simulink model "full_maneuver_platoon"  (R2022a)
settings: Solver=ode23t  StartTime=0.0  StopTime=300  FixedStep=0.1  MaxStep=0.01  RelTol=1e-3
InitFcn:
  | totalVehicles = 7;
  | if exist('vehStatesBus', 'var')==0
  | load vehBuses
  | end
  | if exist('vehErrorsBus', 'var')==0
  | load vehBuses
  | end
libraries: simulink x80, powerlib_meascontrol x16, autolibshared x7, dspsigops x4
(part 3 of 9)

== system full_maneuver_platoon/p1/CACC origin lane ==
  ego : Inport
  leader : Inport  Port=2
  referenceSpeed : Inport  Port=3
  leaderChange : Inport  Port=4
  extraSpaceFlag : Inport  Port=5
  Bus Selector : BusSelector  OutputSignals=u
  Compute Errors : Subsystem
  Constant : Constant  Value=0
  Constant1 : Constant  Value=1.2*freeFlowVel
  Define Desired Distance : Subsystem
  Demux : Demux  Outputs=2
  NOT : Logic  Operator=NOT  IconShape=distinctive  AllPortsSameDT=off  OutDataTypeStr=boolean
  NOT1 : Logic  Operator=NOT  IconShape=distinctive  AllPortsSameDT=off  OutDataTypeStr=boolean
  Rate Limiter : RateLimiter  RisingSlewLimit=maxJerk  FallingSlewLimit=minJerk  SampleTimeMode=inherited
  Rate Limiter1 : RateLimiter  RisingSlewLimit=maxComfJerk  FallingSlewLimit=minComfJerk  SampleTimeMode=inherited
  Switch : Switch  Criteria=u2 > Threshold  SaturateOnIntegerOverflow=off  InputSameDT=off
  Switch1 : Switch  Criteria=u2 > Threshold  SaturateOnIntegerOverflow=off  InputSameDT=off
  Veh Following : Subsystem  TreatAsAtomicUnit=on
  Velocity Control : Subsystem  TreatAsAtomicUnit=on
  Velocity Error : Subsystem
  comf saturation : Saturate  UpperLimit=maxComfAccel  LowerLimit=minComfAccel
  errorScope : Scope  NumInputPorts=2
  safe saturation : Saturate  UpperLimit=maxAcceleration  LowerLimit=minAcceleration
  switch free flow : Subsystem
  veh foll state : Scope  NumInputPorts=2
  errors : Outport
  gap : Outport  Port=2
  u : Outport  Port=3
  real veh foll state : Outport  Port=4
  wires:
  Compute Errors/3("gap ") -> gap/1, switch free flow/3(gap)
  Compute Errors/1(errors) -> Veh Following/1(errors), Demux/1, errors/1, switch free flow/1(errors)
  Switch1/1 -> u/1
  Demux/1 -> errorScope/1
  Demux/2 -> errorScope/2
  NOT1/1 -> Velocity Control/3(integralReset)
  NOT/1 -> Velocity Error/3(filterReset)
  Constant1/1 -> switch free flow/6(vRef)
  extraSpaceFlag/1 -> Define Desired Distance/1(extraSpaceFlag)
  switch free flow/1(inRange) -> NOT/1, NOT1/1, real veh foll state/1, veh foll state/1, Switch/2, Veh Following/5(inRange)
  Velocity Error/1(ev) -> Velocity Control/1(ev)
  Velocity Error/2(ea) -> Velocity Control/2(ea)
  leaderChange/1 -> Veh Following/4(leaderChange)
  Veh Following/1(u) -> Switch/1
  Constant/1 -> Compute Errors/5(velFilterReset)
  leader/1 -> Compute Errors/2(leader)
  comf saturation/1 -> Rate Limiter1/1
  safe saturation/1 -> Rate Limiter/1
  Rate Limiter/1 -> Switch1/1  "sat(u)"
  Switch/1 -> comf saturation/1, safe saturation/1, veh foll state/2
  Rate Limiter1/1 -> Switch1/3  "sat(u)"
  ego/1 -> Velocity Error/1(ego), Bus Selector/1, Compute Errors/1(ego)
  Velocity Control/1(u) -> Switch/3
  referenceSpeed/1 -> Velocity Error/2(velRef)
  Compute Errors/4(unsafeFlag) -> Switch1/2
  Bus Selector/1 -> Veh Following/3(realInput)  "<u>"
  Compute Errors/2(errorsDot) -> switch free flow/2(errorsDot), Veh Following/2(errorsDot)
  Define Desired Distance/1(h) -> switch free flow/4(h), Compute Errors/3(h)
  Define Desired Distance/2(d0) -> switch free flow/5(d0), Compute Errors/4(d0)

== system full_maneuver_platoon/p1/Check if Gap is Closed ==
  In1 : Inport
  AND : Logic  Inputs=1  IconShape=distinctive  AllPortsSameDT=off  OutDataTypeStr=boolean
  Abs2 : Abs  SaturateOnIntegerOverflow=off
  Compare To Constant2 : simulink/Logic and Bit Operations/Compare To Constant  relop=<=  const=1  OutDataTypeStr=boolean
  Mux : Mux  Inputs=2
  Transport Delay2 : TransportDelay
  Out1 : Outport
  wires:
  Transport Delay2/1 -> Mux/1
  Abs2/1 -> Compare To Constant2/1
  Compare To Constant2/1 -> AND/1
  Mux/1 -> Abs2/1
  In1/1 -> Transport Delay2/1, Mux/2
  AND/1 -> Out1/1

== system full_maneuver_platoon/p1/Find Leader ==
  ego : Inport
  all : Inport  Port=2
  canStartLaneChange : Inport  Port=3
  laneChangeDone : Inport  Port=4
  Detect Change : simulink/Logic and Bit Operations/Detect Change  vinit=0  OutDataTypeStr=boolean
  NOT : Logic  Operator=NOT  IconShape=distinctive  AllPortsSameDT=off  OutDataTypeStr=boolean
  OR : Logic  Operator=OR  IconShape=distinctive  AllPortsSameDT=off  OutDataTypeStr=boolean
  Selector : Selector  InputPortWidth=totalVehicles+1  IndexOptions=Index vector (port)  Indices=[1]  OutputSizes=1
  Subsystem : Subsystem
  Vector Concatenate : Concatenate
  farAwayVeh : Subsystem
  realLeaderIdx : Scope
  leader : Outport  VectorParamsAs1DForOutWhenUnconnected=off
  leaderChange : Outport  Port=2  VectorParamsAs1DForOutWhenUnconnected=off
  wires:
  Vector Concatenate/1 -> Selector/1
  farAwayVeh/1(Out1) -> Vector Concatenate/2
  Subsystem/1(idx) -> Detect Change/1, Selector/2, realLeaderIdx/1
  NOT/1 -> OR/1
  canStartLaneChange/1 -> NOT/1
  OR/1 -> Subsystem/Enable  "isLaneChanging"
  all/1 -> Subsystem/2(all), Vector Concatenate/1
  ego/1 -> farAwayVeh/1(ego), Subsystem/1(ego)
  laneChangeDone/1 -> OR/2
  Selector/1 -> leader/1
  Detect Change/1 -> leaderChange/1

== system full_maneuver_platoon/p1/Lane Change Strategy ==
  note: 1) Add Subsystem or Model blocks as valid variant choices.
      | 2) You cannot connect blocks at this level. At simulation, connectivity is automatically
      | determined, based on the active variant and port name matching.
  gapRequest : Inport
  lcFlag : Inport  Port=2
  positionInPlatoon : Inport  Port=3
  platoonStates : Inport  Port=4
  isLaneChangeSafe : Inport  Port=5
  isLaneChangeDone : Inport  Port=6
  isGapClosed : Inport  Port=7
  realCACCstate : Inport  Port=8
  Strategy 1: synchronous : Subsystem  VariantControl=synchronous
  Strategy 2: leader first : Subsystem  VariantControl=leaderFirst
  Strategy 3: last first : Subsystem  VariantControl=lastFirst
  Strategy 4: leader first invert : Subsystem  VariantControl=leaderFirstInvert
  maneuverState : Outport
  mustIncreaseGap : Outport  Port=2
  canStartLaneChange : Outport  Port=3
  hasVirtualLeader : Outport  Port=4
  virtualLeaderIdx : Outport  Port=5
  virtualFollowerIdx : Outport  Port=6

== system full_maneuver_platoon/p1/Lateral Control ==
  measuredStates : Inport
  yRef : Inport  Port=2
  Demux2 : Demux
  Full State Observer : Subsystem  Commented=on
  Gain : Gain  Gain=5
  Gain1 : Gain  Gain=Klat  Multiplication=Matrix(K*u)
  Integrator : Integrator  InitialCondition=y0
  Pad : dspsigops/Pad  padAlong=Columns  dimsToPad=1  valSrc=Specify via dialog  padVal=0  spec=Output size  padNumOutRowsSpecMethod=User-specified  numOutRows=4  padNumOutColsSpecMethod=User-specified  numOutCols=1  isVarDimsMode=off  padBeginning=0  padEnd=0  outSizeMode=User-specified  outSize=1  padSigAt=End  trunc_flag=None  roundingMode=Floor  overflowMode=off  truncOrWrapMode=Truncate  wrap_flag=None
      settings: SourceProductBaseCode=DS
  Rate Limiter : RateLimiter  RisingSlewLimit=maxDeltaDot  FallingSlewLimit=-maxDeltaDot  SampleTimeMode=inherited
  Saturation : Saturate  UpperLimit=maxDelta  LowerLimit=-maxDelta
  Saturation1 : Saturate  UpperLimit=2  LowerLimit=-2
  Scope : Scope  NumInputPorts=4
  Scope1 : Scope  NumInputPorts=2
  Selector : Selector  InputPortWidth=4  IndexOptions=Index vector (dialog)  Indices=[1]  OutputSizes=1
  Sum : Sum  Inputs=|+-
  Sum2 : Sum  Inputs=|+-
  delta : Outport  VectorParamsAs1DForOutWhenUnconnected=off
  ey : Outport  Port=2  VectorParamsAs1DForOutWhenUnconnected=off
  wires:
  Selector/1 -> ey/1
  Saturation1/1 -> Integrator/1
  Gain/1 -> Saturation1/1
  measuredStates/1 -> Sum/2, Demux2/1, Full State Observer/1(measuredOutputs)  "estStates"
  yRef/1 -> Sum2/1
  Demux2/3 -> Scope/3
  Saturation/1 -> Rate Limiter/1
  Sum2/1 -> Gain/1
  Demux2/2 -> Scope/2
  Demux2/4 -> Scope/4
  Pad/1 -> Sum/1
  Sum/1 -> Gain1/1, Selector/1
  Gain1/1 -> Saturation/1, Scope1/2
  Integrator/1 -> Pad/1, Sum2/2
  Demux2/1 -> Scope/1
  Rate Limiter/1 -> delta/1, Scope1/1, Full State Observer/2(delta)  "delta"

== system full_maneuver_platoon/p1/Subsystem ==
  real u : Inport
  real CACC state : Inport  Port=2
  virtual u : Inport  Port=3
  virtual CACC active : Inport  Port=4
  AND : Logic  IconShape=distinctive  AllPortsSameDT=off  OutDataTypeStr=boolean
  Min : MinMax  Inputs=2
  NOT : Logic  Operator=NOT  IconShape=distinctive  AllPortsSameDT=off  OutDataTypeStr=boolean
  Switch : Switch  Criteria=u2 ~= 0  SaturateOnIntegerOverflow=off  InputSameDT=off
  possible inputs : Scope  NumInputPorts=2
  u : Outport
  wires:
  real u/1 -> Min/1, possible inputs/1
  virtual u/1 -> Switch/1, Min/2, possible inputs/2
  Min/1 -> Switch/3
  real CACC state/1 -> NOT/1
  NOT/1 -> AND/1
  virtual CACC active/1 -> AND/2
  AND/1 -> Switch/2
  Switch/1 -> u/1

== system full_maneuver_platoon/p1/Virtual Follower Error ==
  all : Inport
  virtualFollowerIdx : Inport  Port=2
  Enable : EnablePort
  Bus Selector : BusSelector  OutputSignals=egVirtual,evVirtual
  Mux : Mux  Inputs=2
  Scope : Scope
  Selector1 : Selector  InputPortWidth=totalVehicles  IndexOptions=Index vector (port)  Indices=[1]  OutputSizes=1
  virtual follower scope : Scope  NumInputPorts=2
  virtualError : Outport  InitialOutput=[0; 0]
  wires:
  all/1 -> Selector1/1
  virtualFollowerIdx/1 -> Scope/1, Selector1/2
  Mux/1 -> virtualError/1
  Selector1/1 -> Bus Selector/1
  Bus Selector/1 -> Mux/1, virtual follower scope/1  "<egVirtual>"
  Bus Selector/2 -> Mux/2, virtual follower scope/2  "<evVirtual>"

== system full_maneuver_platoon/p1/lateral steady state ==
  e : Inport
  AND : Logic  IconShape=distinctive  AllPortsSameDT=off  OutDataTypeStr=boolean
  Abs2 : Abs  SaturateOnIntegerOverflow=off
  Compare To Constant2 : simulink/Logic and Bit Operations/Compare To Constant  relop=<=  const=0.1  OutDataTypeStr=boolean
  Demux : Demux  Outputs=2
  Mux : Mux  Inputs=2
  Transport Delay2 : TransportDelay
  ssFlag : Outport  VectorParamsAs1DForOutWhenUnconnected=off
  wires:
  Demux/2 -> AND/2
  Mux/1 -> Abs2/1
  Compare To Constant2/1 -> Demux/1
  AND/1 -> ssFlag/1
  Transport Delay2/1 -> Mux/1
  Demux/1 -> AND/1
  Abs2/1 -> Compare To Constant2/1
  e/1 -> Mux/2, Transport Delay2/1

== system full_maneuver_platoon/p1/safeErrors ==
  errors : Inport
  AND : Logic  Inputs=1  IconShape=distinctive  AllPortsSameDT=off  OutDataTypeStr=boolean
  Compare To Constant4 : simulink/Logic and Bit Operations/Compare To Constant  relop=>=  const=-0.1  OutDataTypeStr=boolean
  safetyFlag : Outport  VectorParamsAs1DForOutWhenUnconnected=off
  wires:
  Compare To Constant4/1 -> AND/1
  errors/1 -> Compare To Constant4/1
  AND/1 -> safetyFlag/1

== system full_maneuver_platoon/p1/safeErrors1 ==
  errors : Inport
  AND : Logic  Inputs=1  IconShape=distinctive  AllPortsSameDT=off  OutDataTypeStr=boolean
  Compare To Constant4 : simulink/Logic and Bit Operations/Compare To Constant  relop=>=  const=-0.3  OutDataTypeStr=boolean
  safetyFlag : Outport  VectorParamsAs1DForOutWhenUnconnected=off
  wires:
  Compare To Constant4/1 -> AND/1
  errors/1 -> Compare To Constant4/1
  AND/1 -> safetyFlag/1

== system full_maneuver_platoon/p1/safeErrors2 ==
  errors : Inport
  AND : Logic  Inputs=1  IconShape=distinctive  AllPortsSameDT=off  OutDataTypeStr=boolean
  Compare To Constant4 : simulink/Logic and Bit Operations/Compare To Constant  relop=>=  const=-0.3  OutDataTypeStr=boolean
  safetyFlag : Outport  VectorParamsAs1DForOutWhenUnconnected=off
  wires:
  Compare To Constant4/1 -> AND/1
  AND/1 -> safetyFlag/1
  errors/1 -> Compare To Constant4/1

== system full_maneuver_platoon/p1/states routing ==
  delta : Inport
  Info : Inport  Port=2
  u : Inport  Port=3
  realError : Inport  Port=4
  virtualError : Inport  Port=5
  IatError : Inport  Port=6
  Bus Creator : BusCreator  Inputs=12  OutDataTypeStr=Bus: vehStatesBus  NonVirtualBus=on
      settings: InheritFromInputs=off
  Bus Selector : BusSelector  OutputSignals=BdyFrm.Cg.Vel.ydot,BdyFrm.Cg.AngVel.r,InertFrm.RearAxl.Disp.X,InertFrm.Cg.Disp.Y,InertFrm.RearAxl.Vel.Xdot,BdyFrm.Cg.Acc.xddot,InertFrm.Cg.Ang.psi
  Demux : Demux  Outputs=2
  Demux1 : Demux  Outputs=2
  Mux : Mux
  latStates : Outport
  observedStates : Outport  Port=2
  wires:
  Info/1 -> Bus Selector/1
  Bus Selector/3 -> Bus Creator/1  "<X>"
  Bus Selector/4 -> Bus Creator/2, Mux/1  "<Y>"
  Bus Selector/5 -> Bus Creator/3  "<Xdot>"
  Bus Selector/6 -> Bus Creator/4  "<xddot>"
  Bus Selector/7 -> Mux/3, Bus Creator/5  "<psi>"
  u/1 -> Bus Creator/6
  delta/1 -> Bus Creator/7
  Mux/1 -> latStates/1
  Bus Selector/1 -> Mux/2  "<ydot>"
  Bus Selector/2 -> Mux/4  "<r>"
  Bus Creator/1 -> observedStates/1
  realError/1 -> Demux/1
  virtualError/1 -> Demux1/1
  Demux/1 -> Bus Creator/8
  Demux/2 -> Bus Creator/9
  Demux1/1 -> Bus Creator/10
  Demux1/2 -> Bus Creator/11
  IatError/1 -> Bus Creator/12

== system full_maneuver_platoon/p1/steadyState ==
  u : Inport
  AND : Logic  Inputs=1  IconShape=distinctive  AllPortsSameDT=off  OutDataTypeStr=boolean
  Abs2 : Abs  SaturateOnIntegerOverflow=off
  Compare To Constant2 : simulink/Logic and Bit Operations/Compare To Constant  relop=<=  const=0.2  OutDataTypeStr=boolean
  Mux : Mux  Inputs=2
  Transport Delay2 : TransportDelay
  ssFlag : Outport  VectorParamsAs1DForOutWhenUnconnected=off
  wires:
  Compare To Constant2/1 -> AND/1
  u/1 -> Transport Delay2/1, Mux/2
  Abs2/1 -> Compare To Constant2/1
  Transport Delay2/1 -> Mux/1
  AND/1 -> ssFlag/1
  Mux/1 -> Abs2/1

== system full_maneuver_platoon/p2/CACC destination lane ==
  ego : Inport
  all : Inport  Port=2
  virtualLeaderIdx : Inport  Port=3
  extraSpace : Inport  Port=4
  Enable : EnablePort
  Demux : Demux  Outputs=2
  Detect Change : simulink/Logic and Bit Operations/Detect Change  vinit=0  OutDataTypeStr=boolean
  Scope virtualLeaderIdx : Scope
  Selector : Selector  InputPortWidth=totalVehicles  IndexOptions=Index vector (port)  Indices=[1]  OutputSizes=1
  Subsystem : Subsystem  Commented=through
  Virtual Vehicle Following : Subsystem  TreatAsAtomicUnit=on
  virtual error scope : Scope  NumInputPorts=2
  u : Outport  OutputWhenDisabled=reset  InitialOutput=maxAcceleration+1
  virtualErrors : Outport  Port=2  InitialOutput=[0; 0]
  virtualGap : Outport  Port=3  InitialOutput=[0]
  wires:
  Subsystem/1(u smooth) -> u/1
  virtualLeaderIdx/1 -> Detect Change/1, Selector/2, Scope virtualLeaderIdx/1
  all/1 -> Selector/1
  Demux/2 -> virtual error scope/2
  Demux/1 -> virtual error scope/1
  ego/1 -> Virtual Vehicle Following/1(ego)
  Virtual Vehicle Following/1(u) -> Subsystem/1(u)
  Virtual Vehicle Following/3(virtualGap) -> virtualGap/1
  Virtual Vehicle Following/2(virtualErrors) -> virtualErrors/1, Demux/1
  Detect Change/1 -> Virtual Vehicle Following/3(leaderChange)
  Selector/1 -> Virtual Vehicle Following/2(virtualLeader)
  extraSpace/1 -> Virtual Vehicle Following/4(extraSpaceFlag)

== system full_maneuver_platoon/p2/CACC origin lane ==
  ego : Inport
  leader : Inport  Port=2
  referenceSpeed : Inport  Port=3
  leaderChange : Inport  Port=4
  extraSpaceFlag : Inport  Port=5
  Bus Selector : BusSelector  OutputSignals=u
  Compute Errors : Subsystem
  Constant : Constant  Value=0
  Constant1 : Constant  Value=1.2*freeFlowVel
  Define Desired Distance : Subsystem
  Demux : Demux  Outputs=2
  NOT : Logic  Operator=NOT  IconShape=distinctive  AllPortsSameDT=off  OutDataTypeStr=boolean
  NOT1 : Logic  Operator=NOT  IconShape=distinctive  AllPortsSameDT=off  OutDataTypeStr=boolean
  Rate Limiter : RateLimiter  RisingSlewLimit=maxJerk  FallingSlewLimit=minJerk  SampleTimeMode=inherited
  Rate Limiter1 : RateLimiter  RisingSlewLimit=maxComfJerk  FallingSlewLimit=minComfJerk  SampleTimeMode=inherited
  Switch : Switch  Criteria=u2 > Threshold  SaturateOnIntegerOverflow=off  InputSameDT=off
  Switch1 : Switch  Criteria=u2 > Threshold  SaturateOnIntegerOverflow=off  InputSameDT=off
  Veh Following : Subsystem  TreatAsAtomicUnit=on
  Velocity Control : Subsystem  TreatAsAtomicUnit=on
  Velocity Error : Subsystem
  comf saturation : Saturate  UpperLimit=maxComfAccel  LowerLimit=minComfAccel
  errorScope : Scope  NumInputPorts=2
  safe saturation : Saturate  UpperLimit=maxAcceleration  LowerLimit=minAcceleration
  switch free flow : Subsystem
  veh foll state : Scope  NumInputPorts=2
  errors : Outport
  gap : Outport  Port=2
  u : Outport  Port=3
  real veh foll state : Outport  Port=4
  wires:
  Define Desired Distance/2(d0) -> Compute Errors/4(d0), switch free flow/5(d0)
  Define Desired Distance/1(h) -> Compute Errors/3(h), switch free flow/4(h)
  Compute Errors/2(errorsDot) -> Veh Following/2(errorsDot), switch free flow/2(errorsDot)
  Bus Selector/1 -> Veh Following/3(realInput)  "<u>"
  Compute Errors/4(unsafeFlag) -> Switch1/2
  referenceSpeed/1 -> Velocity Error/2(velRef)
  Velocity Control/1(u) -> Switch/3
  ego/1 -> Compute Errors/1(ego), Bus Selector/1, Velocity Error/1(ego)
  Rate Limiter1/1 -> Switch1/3  "sat(u)"
  Switch/1 -> veh foll state/2, safe saturation/1, comf saturation/1
  Rate Limiter/1 -> Switch1/1  "sat(u)"
  safe saturation/1 -> Rate Limiter/1
  comf saturation/1 -> Rate Limiter1/1
  leader/1 -> Compute Errors/2(leader)
  Constant/1 -> Compute Errors/5(velFilterReset)
  Veh Following/1(u) -> Switch/1
  leaderChange/1 -> Veh Following/4(leaderChange)
  Velocity Error/2(ea) -> Velocity Control/2(ea)
  Velocity Error/1(ev) -> Velocity Control/1(ev)
  switch free flow/1(inRange) -> Veh Following/5(inRange), Switch/2, veh foll state/1, real veh foll state/1, NOT1/1, NOT/1
  extraSpaceFlag/1 -> Define Desired Distance/1(extraSpaceFlag)
  Constant1/1 -> switch free flow/6(vRef)
  NOT/1 -> Velocity Error/3(filterReset)
  NOT1/1 -> Velocity Control/3(integralReset)
  Demux/2 -> errorScope/2
  Demux/1 -> errorScope/1
  Switch1/1 -> u/1
  Compute Errors/1(errors) -> switch free flow/1(errors), errors/1, Demux/1, Veh Following/1(errors)
  Compute Errors/3("gap ") -> switch free flow/3(gap), gap/1

== system full_maneuver_platoon/p2/Check if Gap is Closed ==
  In1 : Inport
  AND : Logic  Inputs=1  IconShape=distinctive  AllPortsSameDT=off  OutDataTypeStr=boolean
  Abs2 : Abs  SaturateOnIntegerOverflow=off
  Compare To Constant2 : simulink/Logic and Bit Operations/Compare To Constant  relop=<=  const=1  OutDataTypeStr=boolean
  Mux : Mux  Inputs=2
  Transport Delay2 : TransportDelay
  Out1 : Outport
  wires:
  AND/1 -> Out1/1
  In1/1 -> Mux/2, Transport Delay2/1
  Mux/1 -> Abs2/1
  Compare To Constant2/1 -> AND/1
  Abs2/1 -> Compare To Constant2/1
  Transport Delay2/1 -> Mux/1

== system full_maneuver_platoon/p2/Find Leader ==
  ego : Inport
  all : Inport  Port=2
  canStartLaneChange : Inport  Port=3
  laneChangeDone : Inport  Port=4
  Detect Change : simulink/Logic and Bit Operations/Detect Change  vinit=0  OutDataTypeStr=boolean
  NOT : Logic  Operator=NOT  IconShape=distinctive  AllPortsSameDT=off  OutDataTypeStr=boolean
  OR : Logic  Operator=OR  IconShape=distinctive  AllPortsSameDT=off  OutDataTypeStr=boolean
  Selector : Selector  InputPortWidth=totalVehicles+1  IndexOptions=Index vector (port)  Indices=[1]  OutputSizes=1
  Subsystem : Subsystem
  Vector Concatenate : Concatenate
  farAwayVeh : Subsystem
  realLeaderIdx : Scope
  leader : Outport  VectorParamsAs1DForOutWhenUnconnected=off
  leaderChange : Outport  Port=2  VectorParamsAs1DForOutWhenUnconnected=off
  wires:
  Detect Change/1 -> leaderChange/1
  Selector/1 -> leader/1
  laneChangeDone/1 -> OR/2
  ego/1 -> Subsystem/1(ego), farAwayVeh/1(ego)
  all/1 -> Vector Concatenate/1, Subsystem/2(all)
  OR/1 -> Subsystem/Enable  "isLaneChanging"
  canStartLaneChange/1 -> NOT/1
  NOT/1 -> OR/1
  Subsystem/1(idx) -> realLeaderIdx/1, Selector/2, Detect Change/1
  farAwayVeh/1(Out1) -> Vector Concatenate/2
  Vector Concatenate/1 -> Selector/1

== system full_maneuver_platoon/p2/Lane Change Strategy ==
  note: 1) Add Subsystem or Model blocks as valid variant choices.
      | 2) You cannot connect blocks at this level. At simulation, connectivity is automatically
      | determined, based on the active variant and port name matching.
  gapRequest : Inport
  lcFlag : Inport  Port=2
  positionInPlatoon : Inport  Port=3
  platoonStates : Inport  Port=4
  isLaneChangeSafe : Inport  Port=5
  isLaneChangeDone : Inport  Port=6
  isGapClosed : Inport  Port=7
  realCACCstate : Inport  Port=8
  Strategy 1: synchronous : Subsystem  VariantControl=synchronous
  Strategy 2: leader first : Subsystem  VariantControl=leaderFirst
  Strategy 3: last first : Subsystem  VariantControl=lastFirst
  Strategy 4: leader first invert : Subsystem  VariantControl=leaderFirstInvert
  maneuverState : Outport
  mustIncreaseGap : Outport  Port=2
  canStartLaneChange : Outport  Port=3
  hasVirtualLeader : Outport  Port=4
  virtualLeaderIdx : Outport  Port=5
  virtualFollowerIdx : Outport  Port=6

== system full_maneuver_platoon/p2/Lateral Control ==
  measuredStates : Inport
  yRef : Inport  Port=2
  Demux2 : Demux
  Full State Observer : Subsystem  Commented=on
  Gain : Gain  Gain=5
  Gain1 : Gain  Gain=Klat  Multiplication=Matrix(K*u)
  Integrator : Integrator  InitialCondition=y0
  Pad : dspsigops/Pad  padAlong=Columns  dimsToPad=1  valSrc=Specify via dialog  padVal=0  spec=Output size  padNumOutRowsSpecMethod=User-specified  numOutRows=4  padNumOutColsSpecMethod=User-specified  numOutCols=1  isVarDimsMode=off  padBeginning=0  padEnd=0  outSizeMode=User-specified  outSize=1  padSigAt=End  trunc_flag=None  roundingMode=Floor  overflowMode=off  truncOrWrapMode=Truncate  wrap_flag=None
      settings: SourceProductBaseCode=DS
  Rate Limiter : RateLimiter  RisingSlewLimit=maxDeltaDot  FallingSlewLimit=-maxDeltaDot  SampleTimeMode=inherited
  Saturation : Saturate  UpperLimit=maxDelta  LowerLimit=-maxDelta
  Saturation1 : Saturate  UpperLimit=2  LowerLimit=-2
  Scope : Scope  NumInputPorts=4
  Scope1 : Scope  NumInputPorts=2
  Selector : Selector  InputPortWidth=4  IndexOptions=Index vector (dialog)  Indices=[1]  OutputSizes=1
  Sum : Sum  Inputs=|+-
  Sum2 : Sum  Inputs=|+-
  delta : Outport  VectorParamsAs1DForOutWhenUnconnected=off
  ey : Outport  Port=2  VectorParamsAs1DForOutWhenUnconnected=off
  wires:
  Rate Limiter/1 -> Full State Observer/2(delta), Scope1/1, delta/1  "delta"
  Demux2/1 -> Scope/1
  Integrator/1 -> Sum2/2, Pad/1
  Gain1/1 -> Scope1/2, Saturation/1
  Sum/1 -> Selector/1, Gain1/1
  Pad/1 -> Sum/1
  Demux2/4 -> Scope/4
  Demux2/2 -> Scope/2
  Sum2/1 -> Gain/1
  Saturation/1 -> Rate Limiter/1
  Demux2/3 -> Scope/3
  yRef/1 -> Sum2/1
  measuredStates/1 -> Full State Observer/1(measuredOutputs), Demux2/1, Sum/2  "estStates"
  Gain/1 -> Saturation1/1
  Saturation1/1 -> Integrator/1
  Selector/1 -> ey/1

== system full_maneuver_platoon/p2/Subsystem ==
  real u : Inport
  real CACC state : Inport  Port=2
  virtual u : Inport  Port=3
  virtual CACC active : Inport  Port=4
  AND : Logic  IconShape=distinctive  AllPortsSameDT=off  OutDataTypeStr=boolean
  Min : MinMax  Inputs=2
  NOT : Logic  Operator=NOT  IconShape=distinctive  AllPortsSameDT=off  OutDataTypeStr=boolean
  Switch : Switch  Criteria=u2 ~= 0  SaturateOnIntegerOverflow=off  InputSameDT=off
  possible inputs : Scope  NumInputPorts=2
  u : Outport
  wires:
  Switch/1 -> u/1
  AND/1 -> Switch/2
  virtual CACC active/1 -> AND/2
  NOT/1 -> AND/1
  real CACC state/1 -> NOT/1
  Min/1 -> Switch/3
  virtual u/1 -> possible inputs/2, Min/2, Switch/1
  real u/1 -> possible inputs/1, Min/1

== system full_maneuver_platoon/p2/Virtual Follower Error ==
  all : Inport
  virtualFollowerIdx : Inport  Port=2
  Enable : EnablePort
  Bus Selector : BusSelector  OutputSignals=egVirtual,evVirtual
  Mux : Mux  Inputs=2
  Scope : Scope
  Selector1 : Selector  InputPortWidth=totalVehicles  IndexOptions=Index vector (port)  Indices=[1]  OutputSizes=1
  virtual follower scope : Scope  NumInputPorts=2
  virtualError : Outport  InitialOutput=[0; 0]
  wires:
  Bus Selector/2 -> virtual follower scope/2, Mux/2  "<evVirtual>"
  Bus Selector/1 -> virtual follower scope/1, Mux/1  "<egVirtual>"
  Selector1/1 -> Bus Selector/1
  Mux/1 -> virtualError/1
  virtualFollowerIdx/1 -> Selector1/2, Scope/1
  all/1 -> Selector1/1

== system full_maneuver_platoon/p2/lateral steady state ==
  e : Inport
  AND : Logic  IconShape=distinctive  AllPortsSameDT=off  OutDataTypeStr=boolean
  Abs2 : Abs  SaturateOnIntegerOverflow=off
  Compare To Constant2 : simulink/Logic and Bit Operations/Compare To Constant  relop=<=  const=0.1  OutDataTypeStr=boolean
  Demux : Demux  Outputs=2
  Mux : Mux  Inputs=2
  Transport Delay2 : TransportDelay
  ssFlag : Outport  VectorParamsAs1DForOutWhenUnconnected=off
  wires:
  e/1 -> Transport Delay2/1, Mux/2
  Abs2/1 -> Compare To Constant2/1
  Demux/1 -> AND/1
  Transport Delay2/1 -> Mux/1
  AND/1 -> ssFlag/1
  Compare To Constant2/1 -> Demux/1
  Mux/1 -> Abs2/1
  Demux/2 -> AND/2

== system full_maneuver_platoon/p2/safeErrors ==
  errors : Inport
  AND : Logic  Inputs=1  IconShape=distinctive  AllPortsSameDT=off  OutDataTypeStr=boolean
  Compare To Constant4 : simulink/Logic and Bit Operations/Compare To Constant  relop=>=  const=-0.1  OutDataTypeStr=boolean
  safetyFlag : Outport  VectorParamsAs1DForOutWhenUnconnected=off
  wires:
  AND/1 -> safetyFlag/1
  errors/1 -> Compare To Constant4/1
  Compare To Constant4/1 -> AND/1

== system full_maneuver_platoon/p2/safeErrors1 ==
  errors : Inport
  AND : Logic  Inputs=1  IconShape=distinctive  AllPortsSameDT=off  OutDataTypeStr=boolean
  Compare To Constant4 : simulink/Logic and Bit Operations/Compare To Constant  relop=>=  const=-0.3  OutDataTypeStr=boolean
  safetyFlag : Outport  VectorParamsAs1DForOutWhenUnconnected=off
  wires:
  AND/1 -> safetyFlag/1
  errors/1 -> Compare To Constant4/1
  Compare To Constant4/1 -> AND/1

== system full_maneuver_platoon/p2/safeErrors2 ==
  errors : Inport
  AND : Logic  Inputs=1  IconShape=distinctive  AllPortsSameDT=off  OutDataTypeStr=boolean
  Compare To Constant4 : simulink/Logic and Bit Operations/Compare To Constant  relop=>=  const=-0.3  OutDataTypeStr=boolean
  safetyFlag : Outport  VectorParamsAs1DForOutWhenUnconnected=off
  wires:
  errors/1 -> Compare To Constant4/1
  AND/1 -> safetyFlag/1
  Compare To Constant4/1 -> AND/1

== system full_maneuver_platoon/p2/states routing ==
  delta : Inport
  Info : Inport  Port=2
  u : Inport  Port=3
  realError : Inport  Port=4
  virtualError : Inport  Port=5
  IatError : Inport  Port=6
  Bus Creator : BusCreator  Inputs=12  OutDataTypeStr=Bus: vehStatesBus  NonVirtualBus=on
      settings: InheritFromInputs=off
  Bus Selector : BusSelector  OutputSignals=BdyFrm.Cg.Vel.ydot,BdyFrm.Cg.AngVel.r,InertFrm.RearAxl.Disp.X,InertFrm.Cg.Disp.Y,InertFrm.RearAxl.Vel.Xdot,BdyFrm.Cg.Acc.xddot,InertFrm.Cg.Ang.psi
  Demux : Demux  Outputs=2
  Demux1 : Demux  Outputs=2
  Mux : Mux
  latStates : Outport
  observedStates : Outport  Port=2
  wires:
  IatError/1 -> Bus Creator/12
  Demux1/2 -> Bus Creator/11
  Demux1/1 -> Bus Creator/10
  Demux/2 -> Bus Creator/9
  Demux/1 -> Bus Creator/8
  virtualError/1 -> Demux1/1
  realError/1 -> Demux/1
  Bus Creator/1 -> observedStates/1
  Bus Selector/2 -> Mux/4  "<r>"
  Bus Selector/1 -> Mux/2  "<ydot>"
  Mux/1 -> latStates/1
  delta/1 -> Bus Creator/7
  u/1 -> Bus Creator/6
  Bus Selector/7 -> Bus Creator/5, Mux/3  "<psi>"
  Bus Selector/6 -> Bus Creator/4  "<xddot>"
  Bus Selector/5 -> Bus Creator/3  "<Xdot>"
  Bus Selector/4 -> Mux/1, Bus Creator/2  "<Y>"
  Bus Selector/3 -> Bus Creator/1  "<X>"
  Info/1 -> Bus Selector/1

== system full_maneuver_platoon/p2/steadyState ==
  u : Inport
  AND : Logic  Inputs=1  IconShape=distinctive  AllPortsSameDT=off  OutDataTypeStr=boolean
  Abs2 : Abs  SaturateOnIntegerOverflow=off
  Compare To Constant2 : simulink/Logic and Bit Operations/Compare To Constant  relop=<=  const=0.2  OutDataTypeStr=boolean
  Mux : Mux  Inputs=2
  Transport Delay2 : TransportDelay
  ssFlag : Outport  VectorParamsAs1DForOutWhenUnconnected=off
  wires:
  Mux/1 -> Abs2/1
  AND/1 -> ssFlag/1
  Transport Delay2/1 -> Mux/1
  Abs2/1 -> Compare To Constant2/1
  u/1 -> Mux/2, Transport Delay2/1
  Compare To Constant2/1 -> AND/1

== system full_maneuver_platoon/p3/CACC destination lane ==
  ego : Inport
  all : Inport  Port=2
  virtualLeaderIdx : Inport  Port=3
  extraSpace : Inport  Port=4
  Enable : EnablePort
  Demux : Demux  Outputs=2
  Detect Change : simulink/Logic and Bit Operations/Detect Change  vinit=0  OutDataTypeStr=boolean
  Scope virtualLeaderIdx : Scope
  Selector : Selector  InputPortWidth=totalVehicles  IndexOptions=Index vector (port)  Indices=[1]  OutputSizes=1
  Subsystem : Subsystem  Commented=through
  Virtual Vehicle Following : Subsystem  TreatAsAtomicUnit=on
  virtual error scope : Scope  NumInputPorts=2
  u : Outport  OutputWhenDisabled=reset  InitialOutput=maxAcceleration+1
  virtualErrors : Outport  Port=2  InitialOutput=[0; 0]
  virtualGap : Outport  Port=3  InitialOutput=[0]
  wires:
  extraSpace/1 -> Virtual Vehicle Following/4(extraSpaceFlag)
  Selector/1 -> Virtual Vehicle Following/2(virtualLeader)
  Detect Change/1 -> Virtual Vehicle Following/3(leaderChange)
  Virtual Vehicle Following/2(virtualErrors) -> Demux/1, virtualErrors/1
  Virtual Vehicle Following/3(virtualGap) -> virtualGap/1
  Virtual Vehicle Following/1(u) -> Subsystem/1(u)
  ego/1 -> Virtual Vehicle Following/1(ego)
  Demux/1 -> virtual error scope/1
  Demux/2 -> virtual error scope/2
  all/1 -> Selector/1
  virtualLeaderIdx/1 -> Scope virtualLeaderIdx/1, Selector/2, Detect Change/1
  Subsystem/1(u smooth) -> u/1

== system full_maneuver_platoon/p3/CACC origin lane ==
  ego : Inport
  leader : Inport  Port=2
  referenceSpeed : Inport  Port=3
  leaderChange : Inport  Port=4
  extraSpaceFlag : Inport  Port=5
  Bus Selector : BusSelector  OutputSignals=u
  Compute Errors : Subsystem
  Constant : Constant  Value=0
  Constant1 : Constant  Value=1.2*freeFlowVel
  Define Desired Distance : Subsystem
  Demux : Demux  Outputs=2
  NOT : Logic  Operator=NOT  IconShape=distinctive  AllPortsSameDT=off  OutDataTypeStr=boolean
  NOT1 : Logic  Operator=NOT  IconShape=distinctive  AllPortsSameDT=off  OutDataTypeStr=boolean
  Rate Limiter : RateLimiter  RisingSlewLimit=maxJerk  FallingSlewLimit=minJerk  SampleTimeMode=inherited
  Rate Limiter1 : RateLimiter  RisingSlewLimit=maxComfJerk  FallingSlewLimit=minComfJerk  SampleTimeMode=inherited
  Switch : Switch  Criteria=u2 > Threshold  SaturateOnIntegerOverflow=off  InputSameDT=off
  Switch1 : Switch  Criteria=u2 > Threshold  SaturateOnIntegerOverflow=off  InputSameDT=off
  Veh Following : Subsystem  TreatAsAtomicUnit=on
  Velocity Control : Subsystem  TreatAsAtomicUnit=on
  Velocity Error : Subsystem
  comf saturation : Saturate  UpperLimit=maxComfAccel  LowerLimit=minComfAccel
  errorScope : Scope  NumInputPorts=2
  safe saturation : Saturate  UpperLimit=maxAcceleration  LowerLimit=minAcceleration
  switch free flow : Subsystem
  veh foll state : Scope  NumInputPorts=2
  errors : Outport
  gap : Outport  Port=2
  u : Outport  Port=3
  real veh foll state : Outport  Port=4
  wires:
  Compute Errors/3("gap ") -> gap/1, switch free flow/3(gap)
  Compute Errors/1(errors) -> Veh Following/1(errors), Demux/1, errors/1, switch free flow/1(errors)
  Switch1/1 -> u/1
  Demux/1 -> errorScope/1
  Demux/2 -> errorScope/2
  NOT1/1 -> Velocity Control/3(integralReset)
  NOT/1 -> Velocity Error/3(filterReset)
  Constant1/1 -> switch free flow/6(vRef)
  extraSpaceFlag/1 -> Define Desired Distance/1(extraSpaceFlag)
  switch free flow/1(inRange) -> NOT/1, NOT1/1, real veh foll state/1, veh foll state/1, Switch/2, Veh Following/5(inRange)
  Velocity Error/1(ev) -> Velocity Control/1(ev)
  Velocity Error/2(ea) -> Velocity Control/2(ea)
  leaderChange/1 -> Veh Following/4(leaderChange)
  Veh Following/1(u) -> Switch/1
  Constant/1 -> Compute Errors/5(velFilterReset)
  leader/1 -> Compute Errors/2(leader)
  comf saturation/1 -> Rate Limiter1/1
  safe saturation/1 -> Rate Limiter/1
  Rate Limiter/1 -> Switch1/1  "sat(u)"
  Switch/1 -> comf saturation/1, safe saturation/1, veh foll state/2
  Rate Limiter1/1 -> Switch1/3  "sat(u)"
  ego/1 -> Velocity Error/1(ego), Bus Selector/1, Compute Errors/1(ego)
  Velocity Control/1(u) -> Switch/3
  referenceSpeed/1 -> Velocity Error/2(velRef)
  Compute Errors/4(unsafeFlag) -> Switch1/2
  Bus Selector/1 -> Veh Following/3(realInput)  "<u>"
  Compute Errors/2(errorsDot) -> switch free flow/2(errorsDot), Veh Following/2(errorsDot)
  Define Desired Distance/1(h) -> switch free flow/4(h), Compute Errors/3(h)
  Define Desired Distance/2(d0) -> switch free flow/5(d0), Compute Errors/4(d0)

== system full_maneuver_platoon/p3/Check if Gap is Closed ==
  In1 : Inport
  AND : Logic  Inputs=1  IconShape=distinctive  AllPortsSameDT=off  OutDataTypeStr=boolean
  Abs2 : Abs  SaturateOnIntegerOverflow=off
  Compare To Constant2 : simulink/Logic and Bit Operations/Compare To Constant  relop=<=  const=1  OutDataTypeStr=boolean
  Mux : Mux  Inputs=2
  Transport Delay2 : TransportDelay
  Out1 : Outport
  wires:
  Transport Delay2/1 -> Mux/1
  Abs2/1 -> Compare To Constant2/1
  Compare To Constant2/1 -> AND/1
  Mux/1 -> Abs2/1
  In1/1 -> Transport Delay2/1, Mux/2
  AND/1 -> Out1/1

== system full_maneuver_platoon/p3/Find Leader ==
  ego : Inport
  all : Inport  Port=2
  canStartLaneChange : Inport  Port=3
  laneChangeDone : Inport  Port=4
  Detect Change : simulink/Logic and Bit Operations/Detect Change  vinit=0  OutDataTypeStr=boolean
  NOT : Logic  Operator=NOT  IconShape=distinctive  AllPortsSameDT=off  OutDataTypeStr=boolean
  OR : Logic  Operator=OR  IconShape=distinctive  AllPortsSameDT=off  OutDataTypeStr=boolean
  Selector : Selector  InputPortWidth=totalVehicles+1  IndexOptions=Index vector (port)  Indices=[1]  OutputSizes=1
  Subsystem : Subsystem
  Vector Concatenate : Concatenate
  farAwayVeh : Subsystem
  realLeaderIdx : Scope
  leader : Outport  VectorParamsAs1DForOutWhenUnconnected=off
  leaderChange : Outport  Port=2  VectorParamsAs1DForOutWhenUnconnected=off
  wires:
  Vector Concatenate/1 -> Selector/1
  farAwayVeh/1(Out1) -> Vector Concatenate/2
  Subsystem/1(idx) -> Detect Change/1, Selector/2, realLeaderIdx/1
  NOT/1 -> OR/1
  canStartLaneChange/1 -> NOT/1
  OR/1 -> Subsystem/Enable  "isLaneChanging"
  all/1 -> Subsystem/2(all), Vector Concatenate/1
  ego/1 -> farAwayVeh/1(ego), Subsystem/1(ego)
  laneChangeDone/1 -> OR/2
  Selector/1 -> leader/1
  Detect Change/1 -> leaderChange/1

== system full_maneuver_platoon/p3/Lane Change Strategy ==
  note: 1) Add Subsystem or Model blocks as valid variant choices.
      | 2) You cannot connect blocks at this level. At simulation, connectivity is automatically
      | determined, based on the active variant and port name matching.
  gapRequest : Inport
  lcFlag : Inport  Port=2
  positionInPlatoon : Inport  Port=3
  platoonStates : Inport  Port=4
  isLaneChangeSafe : Inport  Port=5
  isLaneChangeDone : Inport  Port=6
  isGapClosed : Inport  Port=7
  realCACCstate : Inport  Port=8
  Strategy 1: synchronous : Subsystem  VariantControl=synchronous
  Strategy 2: leader first : Subsystem  VariantControl=leaderFirst
  Strategy 3: last first : Subsystem  VariantControl=lastFirst
  Strategy 4: leader first invert : Subsystem  VariantControl=leaderFirstInvert
  maneuverState : Outport
  mustIncreaseGap : Outport  Port=2
  canStartLaneChange : Outport  Port=3
  hasVirtualLeader : Outport  Port=4
  virtualLeaderIdx : Outport  Port=5
  virtualFollowerIdx : Outport  Port=6

== system full_maneuver_platoon/p3/Lateral Control ==
  measuredStates : Inport
  yRef : Inport  Port=2
  Demux2 : Demux
  Full State Observer : Subsystem  Commented=on
  Gain : Gain  Gain=5
  Gain1 : Gain  Gain=Klat  Multiplication=Matrix(K*u)
  Integrator : Integrator  InitialCondition=y0
  Pad : dspsigops/Pad  padAlong=Columns  dimsToPad=1  valSrc=Specify via dialog  padVal=0  spec=Output size  padNumOutRowsSpecMethod=User-specified  numOutRows=4  padNumOutColsSpecMethod=User-specified  numOutCols=1  isVarDimsMode=off  padBeginning=0  padEnd=0  outSizeMode=User-specified  outSize=1  padSigAt=End  trunc_flag=None  roundingMode=Floor  overflowMode=off  truncOrWrapMode=Truncate  wrap_flag=None
      settings: SourceProductBaseCode=DS
  Rate Limiter : RateLimiter  RisingSlewLimit=maxDeltaDot  FallingSlewLimit=-maxDeltaDot  SampleTimeMode=inherited
  Saturation : Saturate  UpperLimit=maxDelta  LowerLimit=-maxDelta
  Saturation1 : Saturate  UpperLimit=2  LowerLimit=-2
  Scope : Scope  NumInputPorts=4
  Scope1 : Scope  NumInputPorts=2
  Selector : Selector  InputPortWidth=4  IndexOptions=Index vector (dialog)  Indices=[1]  OutputSizes=1
  Sum : Sum  Inputs=|+-
  Sum2 : Sum  Inputs=|+-
  delta : Outport  VectorParamsAs1DForOutWhenUnconnected=off
  ey : Outport  Port=2  VectorParamsAs1DForOutWhenUnconnected=off
  wires:
  Selector/1 -> ey/1
  Saturation1/1 -> Integrator/1
  Gain/1 -> Saturation1/1
  measuredStates/1 -> Sum/2, Demux2/1, Full State Observer/1(measuredOutputs)  "estStates"
  yRef/1 -> Sum2/1
  Demux2/3 -> Scope/3
  Saturation/1 -> Rate Limiter/1
  Sum2/1 -> Gain/1
  Demux2/2 -> Scope/2
  Demux2/4 -> Scope/4
  Pad/1 -> Sum/1
  Sum/1 -> Gain1/1, Selector/1
  Gain1/1 -> Saturation/1, Scope1/2
  Integrator/1 -> Pad/1, Sum2/2
  Demux2/1 -> Scope/1
  Rate Limiter/1 -> delta/1, Scope1/1, Full State Observer/2(delta)  "delta"

== system full_maneuver_platoon/p3/Subsystem ==
  real u : Inport
  real CACC state : Inport  Port=2
  virtual u : Inport  Port=3
  virtual CACC active : Inport  Port=4
  AND : Logic  IconShape=distinctive  AllPortsSameDT=off  OutDataTypeStr=boolean
  Min : MinMax  Inputs=2
  NOT : Logic  Operator=NOT  IconShape=distinctive  AllPortsSameDT=off  OutDataTypeStr=boolean
  Switch : Switch  Criteria=u2 ~= 0  SaturateOnIntegerOverflow=off  InputSameDT=off
  possible inputs : Scope  NumInputPorts=2
  u : Outport
  wires:
  real u/1 -> Min/1, possible inputs/1
  virtual u/1 -> Switch/1, Min/2, possible inputs/2
  Min/1 -> Switch/3
  real CACC state/1 -> NOT/1
  NOT/1 -> AND/1
  virtual CACC active/1 -> AND/2
  AND/1 -> Switch/2
  Switch/1 -> u/1

== system full_maneuver_platoon/p3/Virtual Follower Error ==
  all : Inport
  virtualFollowerIdx : Inport  Port=2
  Enable : EnablePort
  Bus Selector : BusSelector  OutputSignals=egVirtual,evVirtual
  Mux : Mux  Inputs=2
  Scope : Scope
  Selector1 : Selector  InputPortWidth=totalVehicles  IndexOptions=Index vector (port)  Indices=[1]  OutputSizes=1
  virtual follower scope : Scope  NumInputPorts=2
  virtualError : Outport  InitialOutput=[0; 0]
  wires:
  all/1 -> Selector1/1
  virtualFollowerIdx/1 -> Scope/1, Selector1/2
  Mux/1 -> virtualError/1
  Selector1/1 -> Bus Selector/1
  Bus Selector/1 -> Mux/1, virtual follower scope/1  "<egVirtual>"
  Bus Selector/2 -> Mux/2, virtual follower scope/2  "<evVirtual>"

== system full_maneuver_platoon/p3/lateral steady state ==
  e : Inport
  AND : Logic  IconShape=distinctive  AllPortsSameDT=off  OutDataTypeStr=boolean
  Abs2 : Abs  SaturateOnIntegerOverflow=off
  Compare To Constant2 : simulink/Logic and Bit Operations/Compare To Constant  relop=<=  const=0.1  OutDataTypeStr=boolean
  Demux : Demux  Outputs=2
  Mux : Mux  Inputs=2
  Transport Delay2 : TransportDelay
  ssFlag : Outport  VectorParamsAs1DForOutWhenUnconnected=off
  wires:
  Demux/2 -> AND/2
  Mux/1 -> Abs2/1
  Compare To Constant2/1 -> Demux/1
  AND/1 -> ssFlag/1
  Transport Delay2/1 -> Mux/1
  Demux/1 -> AND/1
  Abs2/1 -> Compare To Constant2/1
  e/1 -> Mux/2, Transport Delay2/1

== system full_maneuver_platoon/p3/safeErrors ==
  errors : Inport
  AND : Logic  Inputs=1  IconShape=distinctive  AllPortsSameDT=off  OutDataTypeStr=boolean
  Compare To Constant4 : simulink/Logic and Bit Operations/Compare To Constant  relop=>=  const=-0.1  OutDataTypeStr=boolean
  safetyFlag : Outport  VectorParamsAs1DForOutWhenUnconnected=off
  wires:
  Compare To Constant4/1 -> AND/1
  errors/1 -> Compare To Constant4/1
  AND/1 -> safetyFlag/1

== system full_maneuver_platoon/p3/safeErrors1 ==
  errors : Inport
  AND : Logic  Inputs=1  IconShape=distinctive  AllPortsSameDT=off  OutDataTypeStr=boolean
  Compare To Constant4 : simulink/Logic and Bit Operations/Compare To Constant  relop=>=  const=-0.3  OutDataTypeStr=boolean
  safetyFlag : Outport  VectorParamsAs1DForOutWhenUnconnected=off
  wires:
  Compare To Constant4/1 -> AND/1
  errors/1 -> Compare To Constant4/1
  AND/1 -> safetyFlag/1

== system full_maneuver_platoon/p3/safeErrors2 ==
  errors : Inport
  AND : Logic  Inputs=1  IconShape=distinctive  AllPortsSameDT=off  OutDataTypeStr=boolean
  Compare To Constant4 : simulink/Logic and Bit Operations/Compare To Constant  relop=>=  const=-0.3  OutDataTypeStr=boolean
  safetyFlag : Outport  VectorParamsAs1DForOutWhenUnconnected=off
  wires:
  Compare To Constant4/1 -> AND/1
  AND/1 -> safetyFlag/1
  errors/1 -> Compare To Constant4/1

== system full_maneuver_platoon/p3/states routing ==
  delta : Inport
  Info : Inport  Port=2
  u : Inport  Port=3
  realError : Inport  Port=4
  virtualError : Inport  Port=5
  IatError : Inport  Port=6
  Bus Creator : BusCreator  Inputs=12  OutDataTypeStr=Bus: vehStatesBus  NonVirtualBus=on
      settings: InheritFromInputs=off
  Bus Selector : BusSelector  OutputSignals=BdyFrm.Cg.Vel.ydot,BdyFrm.Cg.AngVel.r,InertFrm.RearAxl.Disp.X,InertFrm.Cg.Disp.Y,InertFrm.RearAxl.Vel.Xdot,BdyFrm.Cg.Acc.xddot,InertFrm.Cg.Ang.psi
  Demux : Demux  Outputs=2
  Demux1 : Demux  Outputs=2
  Mux : Mux
  latStates : Outport
  observedStates : Outport  Port=2
  wires:
  Info/1 -> Bus Selector/1
  Bus Selector/3 -> Bus Creator/1  "<X>"
  Bus Selector/4 -> Bus Creator/2, Mux/1  "<Y>"
  Bus Selector/5 -> Bus Creator/3  "<Xdot>"
  Bus Selector/6 -> Bus Creator/4  "<xddot>"
  Bus Selector/7 -> Mux/3, Bus Creator/5  "<psi>"
  u/1 -> Bus Creator/6
  delta/1 -> Bus Creator/7
  Mux/1 -> latStates/1
  Bus Selector/1 -> Mux/2  "<ydot>"
  Bus Selector/2 -> Mux/4  "<r>"
  Bus Creator/1 -> observedStates/1
  realError/1 -> Demux/1
  virtualError/1 -> Demux1/1
  Demux/1 -> Bus Creator/8
  Demux/2 -> Bus Creator/9
  Demux1/1 -> Bus Creator/10
  Demux1/2 -> Bus Creator/11
  IatError/1 -> Bus Creator/12

== system full_maneuver_platoon/p3/steadyState ==
  u : Inport
  AND : Logic  Inputs=1  IconShape=distinctive  AllPortsSameDT=off  OutDataTypeStr=boolean
  Abs2 : Abs  SaturateOnIntegerOverflow=off
  Compare To Constant2 : simulink/Logic and Bit Operations/Compare To Constant  relop=<=  const=0.2  OutDataTypeStr=boolean
  Mux : Mux  Inputs=2
  Transport Delay2 : TransportDelay
  ssFlag : Outport  VectorParamsAs1DForOutWhenUnconnected=off
  wires:
  Compare To Constant2/1 -> AND/1
  u/1 -> Transport Delay2/1, Mux/2
  Abs2/1 -> Compare To Constant2/1
  Transport Delay2/1 -> Mux/1
  AND/1 -> ssFlag/1
  Mux/1 -> Abs2/1

== system full_maneuver_platoon/Fd/CACC destination lane/Virtual Vehicle Following ==
  ego : Inport
  virtualLeader : Inport  Port=2
  leaderChange : Inport  Port=3
  extraSpaceFlag : Inport  Port=4
  Bus Selector : BusSelector  OutputSignals=u
  Compute Errors : Subsystem
  Define Desired Distance : Subsystem
  Min Velocity Control : Subsystem  TreatAsAtomicUnit=on
  NOT : Logic  Operator=NOT  IconShape=distinctive  AllPortsSameDT=off  OutDataTypeStr=boolean
  Scope : Scope  NumInputPorts=2
  Switch : Switch  Criteria=u2 > Threshold  SaturateOnIntegerOverflow=off  InputSameDT=off
  Terminator : Terminator
  Velocity Error : Subsystem
  Virtual Leader Following : Subsystem  TreatAsAtomicUnit=on
  comf saturation : Saturate  UpperLimit=maxComfAccel  LowerLimit=minComfAccel
  comf jerk : RateLimiter  RisingSlewLimit=maxComfJerk  FallingSlewLimit=minComfJerk  SampleTimeMode=inherited
  switch min vel : Subsystem
  vMin : Constant  Value=vMin
  u : Outport  InitialOutput=0  VectorParamsAs1DForOutWhenUnconnected=off
  virtualErrors : Outport  Port=2  OutputWhenDisabled=reset  InitialOutput=[0, 0]  VectorParamsAs1DForOutWhenUnconnected=off
  virtualGap : Outport  Port=3  OutputWhenDisabled=reset  InitialOutput=[0]  VectorParamsAs1DForOutWhenUnconnected=off
  wires:
  Switch/1 -> Scope/2, comf saturation/1
  comf jerk/1 -> u/1
  comf saturation/1 -> comf jerk/1
  Bus Selector/1 -> Virtual Leader Following/3(realInput)  "<u>"
  Velocity Error/2(ea) -> Min Velocity Control/2(ea)
  Velocity Error/1(ev) -> Min Velocity Control/1(ev)
  NOT/1 -> Switch/2, Scope/1, Virtual Leader Following/5(inRange)
  switch min vel/1(inRange) -> NOT/1, Min Velocity Control/3(intergralReset), Velocity Error/3(filterReset)
  extraSpaceFlag/1 -> Define Desired Distance/1(extraSpaceFlag)
  Min Velocity Control/1(u) -> Switch/3  "uMinVelControl"
  Compute Errors/3("gap ") -> virtualGap/1, switch min vel/3(gap)
  Virtual Leader Following/1(u) -> Switch/1  "uVehFoll"
  ego/1 -> Compute Errors/1(ego), Bus Selector/1, Velocity Error/1(ego)
  vMin/1 -> switch min vel/6(vRef), Velocity Error/2(velRef)
  Compute Errors/1(errors) -> switch min vel/1(errors), Virtual Leader Following/1(errors), virtualErrors/1
  virtualLeader/1 -> Compute Errors/2(leader)
  leaderChange/1 -> Compute Errors/5(velFilterReset), Virtual Leader Following/4(leaderChange)
  Compute Errors/4(unsafeFlag) -> Terminator/1
  Compute Errors/2(errorsDot) -> Virtual Leader Following/2(errorsDot), switch min vel/2(errorsDot)
  Define Desired Distance/1(h) -> switch min vel/4(h), Compute Errors/3(h)
  Define Desired Distance/2(d0) -> switch min vel/5(d0), Compute Errors/4(d0)

== system full_maneuver_platoon/Fd/CACC origin lane/Controller Real Leader ==
  ego : Inport
  leader : Inport  Port=2
  referenceSpeed : Inport  Port=3
  leaderChange : Inport  Port=4
  extraSpaceFlag : Inport  Port=5
  Bus Selector : BusSelector  OutputSignals=u
  Compute Errors : Subsystem
  Constant : Constant  Value=0
  Constant1 : Constant  Value=1.2*freeFlowVel
  Define Desired Distance : Subsystem
  NOT : Logic  Operator=NOT  IconShape=distinctive  AllPortsSameDT=off  OutDataTypeStr=boolean
  NOT1 : Logic  Operator=NOT  IconShape=distinctive  AllPortsSameDT=off  OutDataTypeStr=boolean
  Rate Limiter : RateLimiter  RisingSlewLimit=maxJerk  FallingSlewLimit=minJerk  SampleTimeMode=inherited
  Rate Limiter1 : RateLimiter  RisingSlewLimit=maxComfJerk  FallingSlewLimit=minComfJerk  SampleTimeMode=inherited
  Switch : Switch  Criteria=u2 > Threshold  SaturateOnIntegerOverflow=off  InputSameDT=off
  Switch1 : Switch  Criteria=u2 > Threshold  SaturateOnIntegerOverflow=off  InputSameDT=off
  Veh Following : Subsystem  TreatAsAtomicUnit=on
  Velocity Control : Subsystem  TreatAsAtomicUnit=on
  Velocity Error : Subsystem
  comf saturation : Saturate  UpperLimit=maxComfAccel  LowerLimit=minComfAccel
  safe saturation : Saturate  UpperLimit=maxAcceleration  LowerLimit=minAcceleration
  switch free flow : Subsystem
  veh foll state : Scope  NumInputPorts=2
  u : Outport  VectorParamsAs1DForOutWhenUnconnected=off
  errors : Outport  Port=2  VectorParamsAs1DForOutWhenUnconnected=off
  gap : Outport  Port=3  VectorParamsAs1DForOutWhenUnconnected=off
  wires:
  NOT1/1 -> Velocity Control/3(integralReset)
  NOT/1 -> Velocity Error/3(filterReset)
  Constant1/1 -> switch free flow/6(vRef)
  extraSpaceFlag/1 -> Define Desired Distance/1(extraSpaceFlag)
  switch free flow/1(inRange) -> Veh Following/5(inRange), Switch/2, veh foll state/1, NOT1/1, NOT/1
  Velocity Error/1(ev) -> Velocity Control/1(ev)
  Velocity Error/2(ea) -> Velocity Control/2(ea)
  leaderChange/1 -> Veh Following/4(leaderChange)
  Veh Following/1(u) -> Switch/1
  Constant/1 -> Compute Errors/5(velFilterReset)
  leader/1 -> Compute Errors/2(leader)
  Compute Errors/1(errors) -> switch free flow/1(errors), Veh Following/1(errors), errors/1
  comf saturation/1 -> Rate Limiter1/1
  safe saturation/1 -> Rate Limiter/1
  Rate Limiter/1 -> Switch1/1  "sat(u)"
  Switch1/1 -> u/1
  Switch/1 -> veh foll state/2, safe saturation/1, comf saturation/1
  Rate Limiter1/1 -> Switch1/3  "sat(u)"
  Compute Errors/3("gap ") -> gap/1, switch free flow/3(gap)
  ego/1 -> Compute Errors/1(ego), Bus Selector/1, Velocity Error/1(ego)
  Velocity Control/1(u) -> Switch/3
  referenceSpeed/1 -> Velocity Error/2(velRef)
  Compute Errors/4(unsafeFlag) -> Switch1/2
  Bus Selector/1 -> Veh Following/3(realInput)  "<u>"
  Compute Errors/2(errorsDot) -> Veh Following/2(errorsDot), switch free flow/2(errorsDot)
  Define Desired Distance/1(h) -> Compute Errors/3(h), switch free flow/4(h)
  Define Desired Distance/2(d0) -> Compute Errors/4(d0), switch free flow/5(d0)

== system full_maneuver_platoon/Fd/Find Leader/Subsystem ==
  ego : Inport
  all : Inport  Port=2
  Enable : EnablePort
  MATLAB Function : MATLAB Function  TreatAsAtomicUnit=on
  idx : Outport  InitialOutput=1  VectorParamsAs1DForOutWhenUnconnected=off
  wires:
  all/1 -> MATLAB Function/2(allVehicles)
  MATLAB Function/1(leaderIdx) -> idx/1
  ego/1 -> MATLAB Function/1(ego)

== system full_maneuver_platoon/Fd/Find Leader/farAwayVeh ==
  ego : Inport  OutDataTypeStr=Bus: vehStatesBus
  Bus Assignment : BusAssignment  AssignedSignals=X
  Bus Selector : BusSelector  OutputSignals=X
  Constant : Constant  Value=1000
  Sum : Sum  Inputs=|++
  Out1 : Outport  OutDataTypeStr=Bus: vehStatesBus  VectorParamsAs1DForOutWhenUnconnected=off
  wires:
  Sum/1 -> Bus Assignment/2  "X"
  Bus Selector/1 -> Sum/1  "<X>"
  Bus Assignment/1 -> Out1/1
  Constant/1 -> Sum/2
  ego/1 -> Bus Selector/1, Bus Assignment/1
